simulink model "PulseCounter"  (R2018a)
settings: Solver=FixedStepAuto  StartTime=0.0  StopTime=10.0  FixedStep=0.5  RelTol=1e-3
settings Model: Creator=Bhaskar  LastModifiedBy=Bhaskar

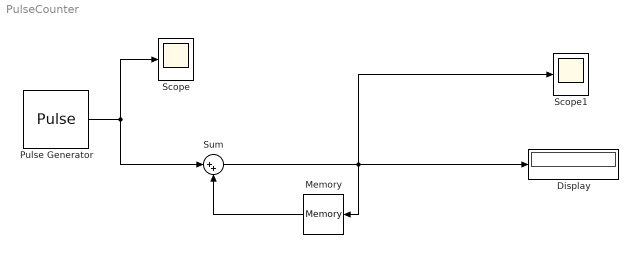
== system PulseCounter ==
  Display : Display
  Memory : Memory
  Pulse Generator : DiscretePulseGenerator  PulseType=Time based  Period=1  PulseWidth=50
  Scope : Scope
  Scope1 : Scope
  Sum : Sum  Inputs=|++
  wires:
  Pulse Generator/1 -> Sum/1, Scope/1
  Memory/1 -> Sum/2
  Sum/1 -> Scope1/1, Display/1, Memory/1
